simulink model "zad_no_2_a"  (R2017b)
settings: Solver=VariableStepAuto  StartTime=0.0  StopTime=10.0  RelTol=1e-3
undefined symbols (not defined in the file): Ini, Tp
settings Model: Creator=micha  LastModifiedBy=micha

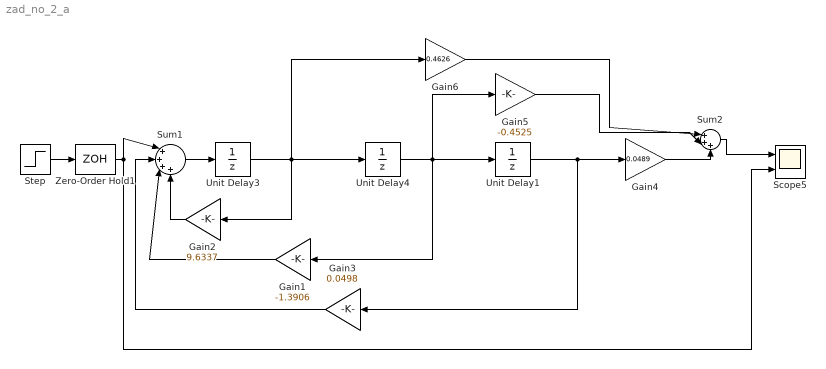
== system zad_no_2_a ==
  Gain1 : Gain  Gain=-1.3906  ParamDataTypeStr=double
  Gain2 : Gain  Gain=9.6337  ParamDataTypeStr=double
  Gain3 : Gain  Gain=0.0498  ParamDataTypeStr=double
  Gain4 : Gain  Gain=0.0489  ParamDataTypeStr=double
  Gain5 : Gain  Gain=-0.4525  ParamDataTypeStr=double
  Gain6 : Gain  Gain=0.4626  ParamDataTypeStr=double
  Scope5 : Scope  NumInputPorts=2
  Step : Step  SampleTime=0
  Sum1 : Sum  Inputs=|++++
  Sum2 : Sum  Inputs=|+++
  Unit Delay1 : UnitDelay  InitialCondition=Ini  SampleTime=Tp
  Unit Delay3 : UnitDelay  InitialCondition=Ini  SampleTime=Tp
  Unit Delay4 : UnitDelay  InitialCondition=Ini  SampleTime=Tp
  Zero-Order Hold1 : ZeroOrderHold  SampleTime=Tp
  wires:
  Unit Delay3/1 -> Gain6/1, Unit Delay4/1, Gain2/1
  Gain6/1 -> Sum2/1
  Gain3/1 -> Sum1/2
  Gain2/1 -> Sum1/4
  Gain4/1 -> Sum2/3
  Zero-Order Hold1/1 -> Scope5/2, Sum1/1
  Gain1/1 -> Sum1/3
  Unit Delay1/1 -> Gain4/1, Gain3/1
  Gain5/1 -> Sum2/2
  Sum1/1 -> Unit Delay3/1
  Unit Delay4/1 -> Gain5/1, Gain1/1, Unit Delay1/1
  Step/1 -> Zero-Order Hold1/1
  Sum2/1 -> Scope5/1
